simulink model "plant"  (R2021b)
settings: Solver=VariableStepAuto  StartTime=0.0  StopTime=10.0  RelTol=1e-3
model workspace (MAT data in the model file):
  c = 0
  k1 = Simulink.Parameter
  k1.Value = 29000
  k1.DataType = 'auto'
  k1.Complexity = 'real'
  k1.Dimensions = [1 1]
  k2 = Simulink.Parameter
  k2.Value = 228000
  k2.DataType = 'auto'
  k2.Complexity = 'real'
  k2.Dimensions = [1 1]
  m1 = Simulink.Parameter
  m1.Value = 380
  m1.DataType = 'auto'
  m1.Complexity = 'real'
  m1.Dimensions = [1 1]
  m2 = Simulink.Parameter
  m2.Value = 31
  m2.DataType = 'auto'
  m2.Complexity = 'real'
  m2.Dimensions = [1 1]
settings Model: Creator=antonio  LastModifiedBy=antonio

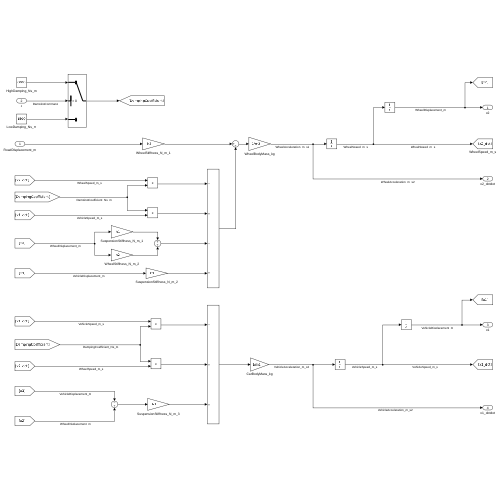
[thumbnail: Simulink's stored preview of the top-level diagram]
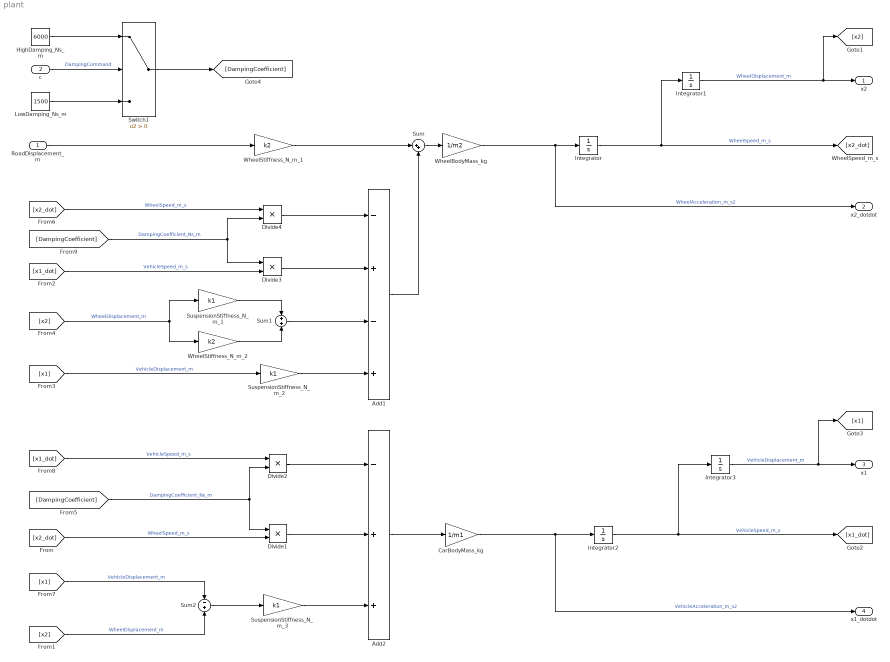
== system plant ==
  RoadDisplacement_m : Inport  OutDataTypeStr=double
  c : Inport  Port=2  OutDataTypeStr=int8
  Add1 : Sum  Inputs=-+-+
  Add2 : Sum  Inputs=-++
  CarBodyMass_kg : Gain  Gain=1/m1
  Divide{1..4} (4 alike) : Product  Inputs=**
  HighDamping_Ns_m : Constant  Value=6000
  Integrator{,1..3} (4 alike) : Integrator
  LowDamping_Ns_m : Constant  Value=1500
  Sum : Sum  Inputs=|++
  Sum1 : Sum
  Sum2 : Sum  Inputs=-+
  SuspensionStiffness_N_m_1 : Gain  Gain=k1
  SuspensionStiffness_N_m_2 : Gain  Gain=k1
  SuspensionStiffness_N_m_3 : Gain  Gain=k1
  Switch1 : Switch  Criteria=u2 > Threshold
  WheelBodyMass_kg : Gain  Gain=1/m2
  WheelStiffness_N_m_1 : Gain  Gain=k2
  WheelStiffness_N_m_2 : Gain  Gain=k2
  x2 : Outport  OutDataTypeStr=double
  x2_dotdot : Outport  Port=2
  x1 : Outport  Port=3  OutDataTypeStr=double
  x1_dotdot : Outport  Port=4
  wires:
  Sum/1 -> WheelBodyMass_kg/1
  Add2/1 -> CarBodyMass_kg/1
  CarBodyMass_kg/1 -> x1_dotdot/1, Integrator2/1  "VehicleAcceleration_m_s2"
  [x1_dot] -> Divide2/1  "VehicleSpeed_m_s"
  Add1/1 -> Sum/2
  WheelBodyMass_kg/1 -> x2_dotdot/1, Integrator/1  "WheelAcceleration_m_s2"
  [x2_dot] -> Divide1/2  "WheelSpeed_m_s"
  Integrator1/1 -> [x2], x2/1  "WheelDisplacement_m"
  WheelStiffness_N_m_1/1 -> Sum/1
  Divide1/1 -> Add2/2
  Divide2/1 -> Add2/1
  Integrator2/1 -> [x1_dot], Integrator3/1  "VehicleSpeed_m_s"
  RoadDisplacement_m/1 -> WheelStiffness_N_m_1/1
  [x1] -> SuspensionStiffness_N_m_2/1  "VehicleDisplacement_m"
  SuspensionStiffness_N_m_3/1 -> Add2/3
  Integrator/1 -> [x2_dot], Integrator1/1  "WheelSpeed_m_s"
  [x2_dot] -> Divide4/1  "WheelSpeed_m_s"
  Divide4/1 -> Add1/1
  Divide3/1 -> Add1/2
  [x1_dot] -> Divide3/2  "VehicleSpeed_m_s"
  SuspensionStiffness_N_m_2/1 -> Add1/4
  [DampingCoefficient] -> Divide1/1, Divide2/2  "DampingCoefficient_Ns_m"
  Sum1/1 -> Add1/3
  [x2] -> WheelStiffness_N_m_2/1, SuspensionStiffness_N_m_1/1  "WheelDisplacement_m"
  WheelStiffness_N_m_2/1 -> Sum1/2
  SuspensionStiffness_N_m_1/1 -> Sum1/1
  c/1 -> Switch1/2  "DampingCommand"
  Switch1/1 -> [DampingCoefficient]
  [DampingCoefficient] -> Divide3/1, Divide4/2  "DampingCoefficient_Ns_m"
  [x1] -> Sum2/1  "VehicleDisplacement_m"
  [x2] -> Sum2/2  "WheelDisplacement_m"
  Sum2/1 -> SuspensionStiffness_N_m_3/1
  Integrator3/1 -> [x1], x1/1  "VehicleDisplacement_m"
  LowDamping_Ns_m/1 -> Switch1/3
  HighDamping_Ns_m/1 -> Switch1/1
